simulink model "Mux4"  (R2023b)
settings: Solver=VariableStepAuto  StartTime=0.0  StopTime=10.0  RelTol=1e-3
settings Model: Creator=jsonm  LastModifiedBy=jsonm

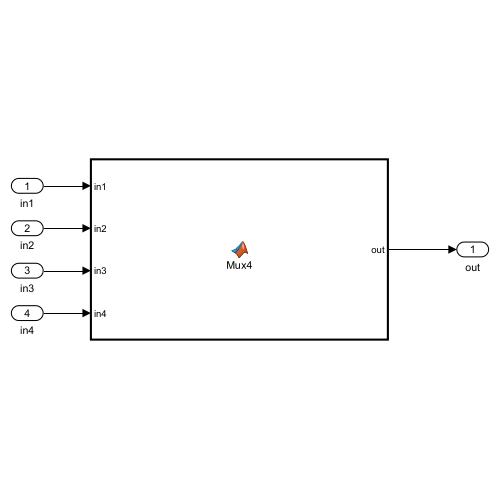
[thumbnail: Simulink's stored preview of the top-level diagram]
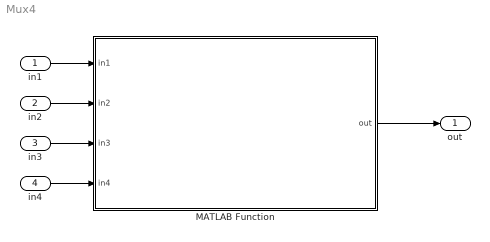
== system Mux4 ==
  in1 : Inport
  in2 : Inport  Port=2
  in3 : Inport  Port=3
  in4 : Inport  Port=4
  MATLAB Function : MATLAB Function  TreatAsAtomicUnit=on
  out : Outport
  wires:
  in1/1 -> MATLAB Function/1(in1)
  in2/1 -> MATLAB Function/2(in2)
  in3/1 -> MATLAB Function/3(in3)
  in4/1 -> MATLAB Function/4(in4)
  MATLAB Function/1(out) -> out/1

== matlab function Mux4/MATLAB Function ==
  data: in1 input; out output; in2 input; in3 input; in4 input
function out = Mux4(in1, in2, in3, in4)

% Method to mux 4 inputs into one of 4 possible outputs based on first
% non-negative input
%
% Written by: Darian Muresan

if nargin < 2
    in2 = -1;
    in3 = -1;
    in4 = -1;
elseif nargin < 3
    in3 = -1;
    in4 = -1;
elseif nargin < 4
    in4 = -1;
end

if in1 >= 0
    out = in1;
elseif in2 >= 0
    out = in2;
elseif in3 >= 0
    out = in3;
elseif in4 >= 0
    out = in4;
else
    out = -1;
end
